simulink model "farenheit_celsius_convertor_rafael_enriquez"  (R2022b)
settings: Solver=VariableStepAuto  StartTime=0.0  StopTime=10.0  RelTol=1e-3
settings Model: Creator=fitir  LastModifiedBy=fitir

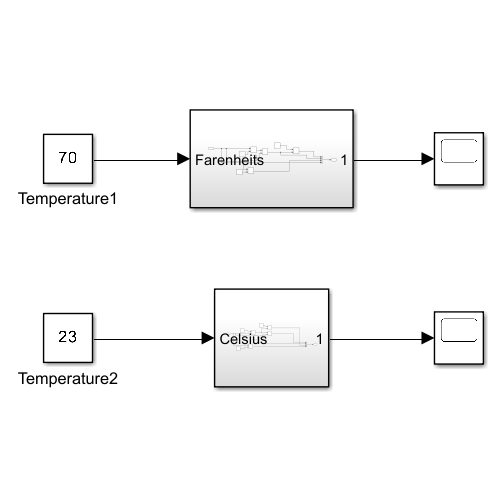
[thumbnail: Simulink's stored preview of the top-level diagram]
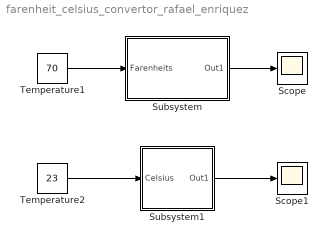
== system farenheit_celsius_convertor_rafael_enriquez ==
  Scope : Scope
  Scope1 : Scope
  Subsystem : Subsystem
  Subsystem1 : Subsystem
  Temperature1 : Constant  Value=70  SampleTime=1
  Temperature2 : Constant  Value=23  SampleTime=1
  wires:
  Temperature1/1 -> Subsystem/1(Farenheits)
  Subsystem/1(Out1) -> Scope/1
  Temperature2/1 -> Subsystem1/1(Celsius)
  Subsystem1/1(Out1) -> Scope1/1

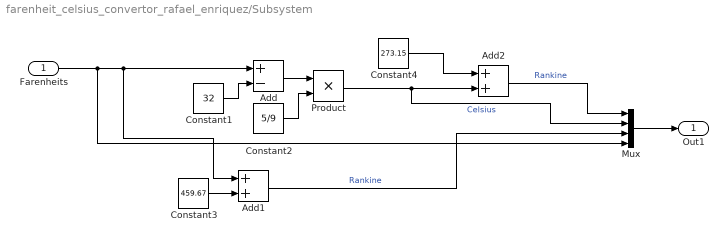
== system farenheit_celsius_convertor_rafael_enriquez/Subsystem ==
  Farenheits : Inport
  Add : Sum  Inputs=+-
  Add1 : Sum
  Add2 : Sum
  Constant1 : Constant  Value=32  SampleTime=1
  Constant2 : Constant  Value=5/9  SampleTime=1
  Constant3 : Constant  Value=459.67  SampleTime=1
  Constant4 : Constant  Value=273.15  SampleTime=1
  Mux : Mux
  Product : Product
  Out1 : Outport
  wires:
  Constant3/1 -> Add1/2
  Add2/1 -> Mux/1  "Rankine"
  Add1/1 -> Mux/3  "Rankine"
  Farenheits/1 -> Mux/4, Add/1, Add1/1
  Product/1 -> Add2/2, Mux/2  "Celsius"
  Constant2/1 -> Product/2
  Add/1 -> Product/1
  Constant4/1 -> Add2/1
  Constant1/1 -> Add/2
  Mux/1 -> Out1/1

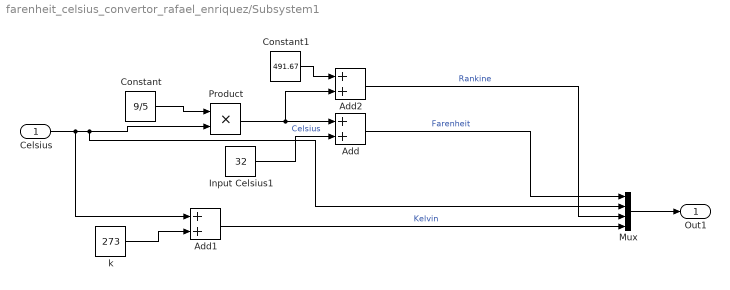
== system farenheit_celsius_convertor_rafael_enriquez/Subsystem1 ==
  Celsius : Inport
  Add : Sum
  Add1 : Sum
  Add2 : Sum
  Constant : Constant  Value=9/5
  Constant1 : Constant  Value=491.67
  Input Celsius1 : Constant  Value=32  SampleTime=1
  Mux : Mux
  Product : Product
  k : Constant  Value=273  SampleTime=1
  Out1 : Outport
  wires:
  Add/1 -> Mux/1  "Farenheit"
  Celsius/1 -> Add1/1, Product/2, Mux/2
  k/1 -> Add1/2
  Product/1 -> Add2/2, Add/1
  Mux/1 -> Out1/1
  Constant/1 -> Product/1
  Add2/1 -> Mux/3  "Rankine"
  Add1/1 -> Mux/4  "Kelvin"
  Input Celsius1/1 -> Add/2  "Celsius"
  Constant1/1 -> Add2/1
